simulink model "siso_4_channel_teleop_discrete_wave_forcePos_noise"  (R2021a)
settings: Solver=FixedStepAuto  StartTime=0.0  StopTime=30  FixedStep=Ts  RelTol=1e-3
values from neighbouring files (symbols this model uses):
  A_kalman = [1 Ts ; 0 1 ]    [assignment6.m]
  Amplitude = 1    [assignment6.m]
  b = 1    [assignment6.m]    (also in lessonParams.m)
  Be = 10    [assignment6.m]    (also in lessonParams.m)
  Bh = 1.5    [assignment6.m]    (also in lessonParams.m)
  Bs = 30    [assignment6.m]
  C_kalman = [1 0]    [assignment6.m]
  delay = 20    [assignment6.m]
  Dh = 2    [assignment6.m]    (also in lessonParams.m)
  Dm = 0    [assignment6.m]
  Ds = 0    [assignment6.m]
  Fc = 0.1    [assignment6.m]    (also in lessonParams.m = 1)
  Flp = 5    [assignment6.m]
  Ih = 0    [assignment6.m]
  Jh = 0    [assignment6.m]    (also in lessonParams.m = 0.05)
  k_h = 2    [assignment6.m]
  Ke = 200    [assignment6.m]    (also in lessonParams.m)
  Kh = 1    [assignment6.m]    (also in lessonParams.m = 0)
  Ks = 40    [assignment6.m]
  Mm = 0.5    [assignment6.m]
  Ms = 2    [assignment6.m]
  noiseVariance = 0.00001    (= 1e-05)    [assignment6.m]
  R = 1    [assignment6.m]
  Ts = 0.001    [assignment6.m]    (also in lessonParams.m)
  xe = 0.65    [assignment6.m]
undefined symbols (not defined in the file or in its folder): B, D, DiscIntNeverNeededParam, Discrete, Time
libraries: simulink x6, ctrlSharedLib x4
settings Model: Creator=fabio  LastModifiedBy=fabio

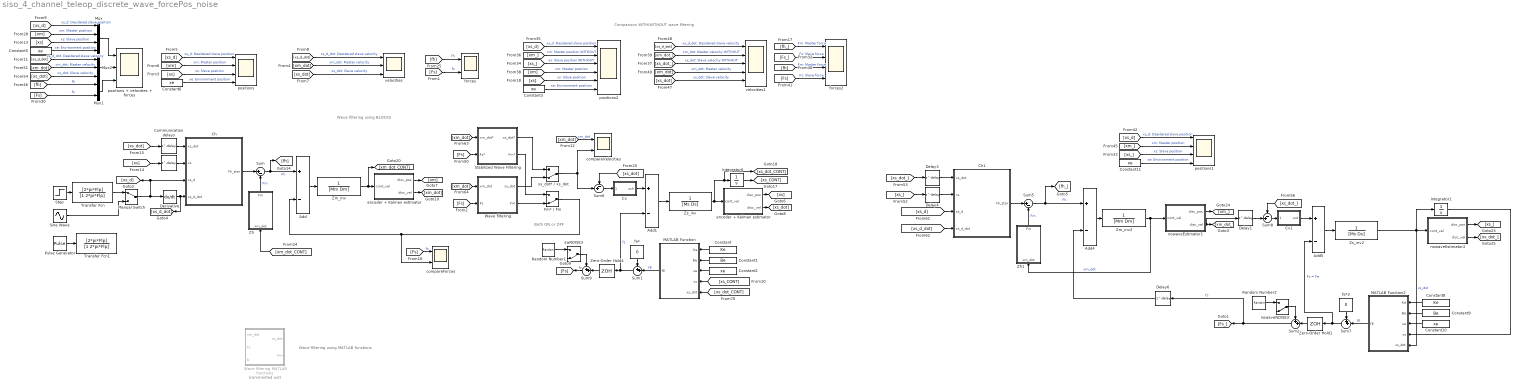
== system siso_4_channel_teleop_discrete_wave_forcePos_noise ==
  note: Both ON or OFF
  note: Wave filtering using BLOCKS
  note: Comparison WITH/WITHOUT wave filtering
  note: Wave filtering using MATLAB functions
  " " : Delay  DelayLength=delay  SampleTime=Ts
  Add{,1,4..5} (4 alike) : Sum  Inputs=+-
  Ch : Subsystem
  Ch1 : Subsystem
  Communication delays : Delay  DelayLength=delay  SampleTime=Ts
  Constant : Constant  Value=Ke
  Constant1 : Constant  Value=Be
  Constant{2..3,5..6,10..11} (6 alike) : Constant  Value=xe
  Constant8 : Constant  Value=Ke
  Constant9 : Constant  Value=Be
  Cv : Subsystem
  Cv1 : Subsystem
  Delay{1,3..4,6} (4 alike) : Delay  DelayLength=delay  SampleTime=Ts
  Derivative : Derivative
  Fm* / Fm : ManualSwitch  CurrentSetting=0
  Integrator1 : Integrator
  Integrator6 : Integrator
  MATLAB Function : MATLAB Function  TreatAsAtomicUnit=on
  MATLAB Function2 : MATLAB Function  TreatAsAtomicUnit=on
  Manual Switch : ManualSwitch
  Mux : Mux
  Mux1 : Mux  Inputs=2
  Mux2 : Mux  Inputs=3
  Pulse Generator : DiscretePulseGenerator  PulseType=Time based  Amplitude=Amplitude  PulseWidth=50  PhaseDelay=1
  Random Number1 : RandomNumber  Variance=noiseVariance  SampleTime=Ts
  Random Number2 : RandomNumber  Variance=noiseVariance  SampleTime=Ts
  Sine Wave : Sin  Amplitude=Amplitude  Frequency=Fc*2*pi  SampleTime=0
  Stabilized Wave Filtering : Subsystem
  Step : Step  After=Amplitude  SampleTime=0
  Sum : Sum  Inputs=|+-
  Sum{1..2,7,9} (4 alike) : Sum  Inputs=++|
  Sum5 : Sum  Inputs=|+-
  Sum6 : Sum  Inputs=-+|
  Sum8 : Sum  Inputs=-+|
  Transfer Fcn : TransferFcn  Numerator=[2*pi*Flp]  Denominator=[1 2*pi*Flp]
  Transfer Fcn1 : TransferFcn  Numerator=[2*pi*Flp]  Denominator=[1 2*pi*Flp]
  Wave filtering : Subsystem
  Wave filtering MATLAB functions : Subsystem  Commented=on
  Zero-Order Hold1 : ZeroOrderHold  SampleTime=Ts
  Zero-Order Hold4 : ZeroOrderHold  SampleTime=Ts
  Zh : Subsystem
  Zh1 : Subsystem
  Zm_inv : TransferFcn  Numerator=[0 1]  Denominator=[Mm Dm]
  Zm_inv2 : TransferFcn  Numerator=[0 1]  Denominator=[Mm Dm]
  Zs_inv : TransferFcn  Numerator=[0 1]  Denominator=[Ms Ds]
  Zs_inv2 : TransferFcn  Numerator=[0 1]  Denominator=[Ms Ds]
  compareForces : Scope  NumInputPorts=2
  compareVelocities : Scope  NumInputPorts=2
  encoder + Kalman estimator : Subsystem
  "encoder + Kalman estimator " : Subsystem
  fe* : Constant  Value=0
  fe*2 : Constant  Value=0
  forces : Scope  NumInputPorts=2
  forces2 : Scope  NumInputPorts=4
  nowaveEstimator1 : Subsystem
  nowaveEstimator2 : Subsystem
  nowaveNOISE3 : ManualSwitch  CurrentSetting=0
  positions : Scope  NumInputPorts=4
  positions + velocities + forces : Scope  NumInputPorts=3
  positions1 : Scope  NumInputPorts=4
  positions2 : Scope  NumInputPorts=6
  swNOISE3 : ManualSwitch  CurrentSetting=0
  velocities : Scope  NumInputPorts=3
  velocities1 : Scope  NumInputPorts=5
  xs_dot* / xs_dot : ManualSwitch  CurrentSetting=0
  wires:
  Zh/1(Fm) -> Sum/2  "Fm"
  Sum/1 -> Add/1, [fh]  "Fh"
  Constant/1 -> MATLAB Function/1(Ke)
  Constant1/1 -> MATLAB Function/2(Be)
  Constant2/1 -> MATLAB Function/3(xe)
  [xs_CONT] -> MATLAB Function/4(xs)
  [xs_dot_CONT] -> MATLAB Function/5(xs_dot)
  MATLAB Function/1(fE) -> Sum1/2  "fE"
  Cv/1(out) -> Add1/1
  Ch/1(Fh_star) -> Sum/1
  [xs_d] -> positions/1  "xs_d: Desidered slave position"
  [xm] -> positions/2  "xm: Master position"
  [xs] -> positions/3  "xs: Slave position"
  [xm_dot] -> velocities/2  "xm_dot: Master velocity"
  [xs_dot] -> velocities/3  "xs_dot: Slave velocity"
  [xs_d_dot] -> velocities/1  "xs_d_dot: Desidered slave velocity"
  Sine Wave/1 -> Manual Switch/2
  Derivative/1 -> [xs_d_dot], Ch/1(xs_d_dot)
  fe*/1 -> Sum1/1
  Step/1 -> Transfer Fcn/1
  Transfer Fcn/1 -> Manual Switch/1
  Manual Switch/1 -> Ch/2(xs_d), [xs_d], Derivative/1
  Constant6/1 -> positions/4  "xe: Environment position"
  [fh] -> forces/1  "fh"
  [Fs] -> forces/2  "fs"
  Pulse Generator/1 -> Transfer Fcn1/1
  [xs_dot] -> Communication delays/1
  Communication delays/1 -> Ch/4(xs_dot)
  " "/1 -> Ch/3(xs)
  [xs_dot] -> Sum6/1
  Sum6/1 -> Cv/1(velErr)
  Wave filtering/1(xs_dot) -> xs_dot* / xs_dot/2
  [Fs] -> Wave filtering/2(Fs)
  [xm_dot] -> compareVelocities/1  "xm_dot"
  [Fs] -> compareForces/1  "fs"
  [xs_d_dot] -> velocities1/1  "xs_d_dot: Desidered slave velocity"
  [xs_dot] -> velocities1/5  "xs_dot: Slave velocity"
  [fh_] -> forces2/1  "Fm: Master force"
  [xs_dot_] -> velocities1/3  "xs_dot: Slave velocity WITHOUT"
  [xm_dot_] -> velocities1/2  "xm_dot: Master velocity WITHOUT"
  [fh] -> forces2/3  "Fm: Master force"
  [xs] -> positions2/5  "xs: Slave position"
  [xs_d] -> positions2/1  "xs_d: Desidered slave position"
  [xm_dot] -> velocities1/4  "xm_dot: Master velocity"
  [Fs_] -> forces2/2  "Fs: Slave force"
  [xs_] -> positions2/3  "xs: Slave position WITHOUT"
  [xm] -> positions2/4  "xm: Master position"
  [xm_] -> positions2/2  "xm: Master position WITHOUT"
  Sum8/1 -> Cv1/1(velErr)
  [xs_dot_] -> Delay3/1
  fe*2/1 -> Sum7/1
  Delay3/1 -> Ch1/4(xs_dot)
  [xs_] -> Delay4/1
  [xs_dot_] -> Sum8/1
  Zh1/1(Fm) -> Sum5/2  "Fm"
  Zm_inv2/1 -> nowaveEstimator1/1(cont_vel), Zh1/1(xm_dot)  "xm_dot"
  Delay4/1 -> Ch1/3(xs)
  Constant9/1 -> MATLAB Function2/2(Be)
  Cv1/1(out) -> Add5/1
  Ch1/1(Fh_star) -> Sum5/1
  MATLAB Function2/1(fE) -> Sum7/2  "fE"
  Add5/1 -> Zs_inv2/1
  Constant10/1 -> MATLAB Function2/3(xe)
  Add4/1 -> Zm_inv2/1
  Constant8/1 -> MATLAB Function2/1(Ke)
  [xs_d] -> Ch1/2(xs_d)
  [xs_d_dot] -> Ch1/1(xs_d_dot)
  Sum5/1 -> [fh_], Add4/1  "Fh"
  [Fs] -> forces2/4  "Fs: Slave force"
  Constant11/1 -> positions1/4  "xe: Environment position"
  [xs_] -> positions1/3  "xs: Slave position"
  [xm_] -> positions1/2  "xm: Master position"
  [xs_d] -> positions1/1  "xs_d: Desidered slave position"
  Delay6/1 -> Add4/2
  nowaveEstimator1/2(disc_vel) -> Delay1/1, [xm_dot_]
  [Fs] -> Stabilized Wave Filtering/2(Fs*)
  xs_dot* / xs_dot/1 -> compareVelocities/2, Sum6/2
  Wave filtering/2(Fm) -> Fm* / Fm/2
  Sum1/1 -> Zero-Order Hold4/1, Add1/2  "fs"
  Zm_inv/1 -> [xm_dot_CONT], encoder + Kalman estimator/1(cont_vel)
  Integrator1/1 -> MATLAB Function2/4(xs)
  Fm* / Fm/1 -> compareForces/2, Add/2
  Zs_inv2/1 -> Integrator1/1, MATLAB Function2/5(xs_dot), nowaveEstimator2/1(cont_vel)  "xs_dot"
  [xm_dot] -> Stabilized Wave Filtering/1(xm_dot*)
  [xm_dot] -> Wave filtering/1(xm_dot)
  Add/1 -> Zm_inv/1
  encoder + Kalman estimator/2(disc_vel) -> [xm_dot]
  "encoder + Kalman estimator "/1(disc_pos) -> [xs]
  Zs_inv/1 -> "encoder + Kalman estimator "/1(cont_vel), [xs_dot_CONT], Integrator6/1
  Integrator6/1 -> [xs_CONT]
  Add1/1 -> Zs_inv/1
  encoder + Kalman estimator/1(disc_pos) -> [xm]
  [xm_dot_CONT] -> Zh/1(xm_dot)
  "encoder + Kalman estimator "/2(disc_vel) -> [xs_dot]
  Random Number1/1 -> swNOISE3/1
  swNOISE3/1 -> Sum9/1
  Sum9/1 -> [Fs]  "fs"
  Zero-Order Hold4/1 -> Sum9/2
  [xs] -> " "/1
  Stabilized Wave Filtering/1(xs_dot*) -> xs_dot* / xs_dot/1
  Stabilized Wave Filtering/2(Fm*) -> Fm* / Fm/1
  nowaveEstimator1/1(disc_pos) -> [xm_]
  nowaveEstimator2/2(disc_vel) -> [xs_dot_]
  nowaveEstimator2/1(disc_pos) -> [xs_]
  Zero-Order Hold1/1 -> Sum2/2
  nowaveNOISE3/1 -> Sum2/1
  Random Number2/1 -> nowaveNOISE3/1
  Sum7/1 -> Add5/2, Zero-Order Hold1/1  "Fs = Fe"
  Sum2/1 -> [Fs_], Delay6/1  "fs"
  Delay1/1 -> Sum8/2
  Constant3/1 -> positions2/6  "xe: Environment position"
  [Fs] -> Mux1/2  "fs"
  [xm] -> Mux/2  "xm: Master position"
  [xs_dot] -> Mux2/3  "xs_dot: Slave velocity"
  [xs] -> Mux/3  "xs: Slave position"
  [xm_dot] -> Mux2/2  "xm_dot: Master velocity"
  [fh] -> Mux1/1  "fh"
  [xs_d] -> Mux/1  "xs_d: Desidered slave position"
  Mux2/1 -> positions + velocities + forces/2
  Mux/1 -> positions + velocities + forces/1
  [xs_d_dot] -> Mux2/1  "xs_d_dot: Desidered slave velocity"
  Mux1/1 -> positions + velocities + forces/3
  Constant5/1 -> Mux/4  "xe: Environment position"

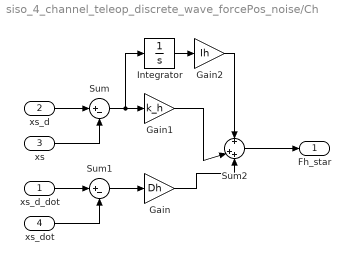
== system siso_4_channel_teleop_discrete_wave_forcePos_noise/Ch ==
  xs_d_dot : Inport
  xs_d : Inport  Port=2
  xs : Inport  Port=3
  xs_dot : Inport  Port=4
  Gain : Gain  Gain=Dh
  Gain1 : Gain  Gain=k_h
  Gain2 : Gain  Gain=Ih
  Integrator : Integrator
  Sum : Sum  Inputs=|+-
  Sum1 : Sum  Inputs=|+-
  Sum2 : Sum  Inputs=+|++
  Fh_star : Outport
  wires:
  Gain1/1 -> Sum2/2
  Sum2/1 -> Fh_star/1
  xs_d/1 -> Sum/1
  xs/1 -> Sum/2
  Sum/1 -> Integrator/1, Gain1/1
  xs_dot/1 -> Sum1/2
  Sum1/1 -> Gain/1
  Gain/1 -> Sum2/3
  xs_d_dot/1 -> Sum1/1
  Integrator/1 -> Gain2/1
  Gain2/1 -> Sum2/1

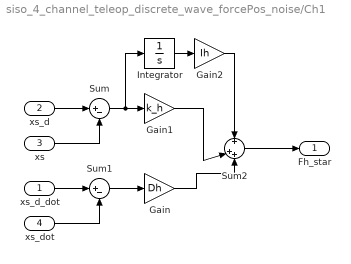
== system siso_4_channel_teleop_discrete_wave_forcePos_noise/Ch1 ==
  xs_d_dot : Inport
  xs_d : Inport  Port=2
  xs : Inport  Port=3
  xs_dot : Inport  Port=4
  Gain : Gain  Gain=Dh
  Gain1 : Gain  Gain=k_h
  Gain2 : Gain  Gain=Ih
  Integrator : Integrator
  Sum : Sum  Inputs=|+-
  Sum1 : Sum  Inputs=|+-
  Sum2 : Sum  Inputs=+|++
  Fh_star : Outport
  wires:
  Gain1/1 -> Sum2/2
  Sum2/1 -> Fh_star/1
  xs_d/1 -> Sum/1
  xs/1 -> Sum/2
  Sum/1 -> Integrator/1, Gain1/1
  xs_dot/1 -> Sum1/2
  Sum1/1 -> Gain/1
  Gain/1 -> Sum2/3
  xs_d_dot/1 -> Sum1/1
  Integrator/1 -> Gain2/1
  Gain2/1 -> Sum2/1

== system siso_4_channel_teleop_discrete_wave_forcePos_noise/Cv ==
  velErr : Inport
  Discrete-Time Integrator : DiscreteIntegrator  SampleTime=-1  ICPrevOutput=DiscIntNeverNeededParam  ICPrevScaledInput=DiscIntNeverNeededParam
  Gain : Gain  Gain=Bs
  Gain1 : Gain  Gain=Ks
  Manual Switch : ManualSwitch
  Sum : Sum  Inputs=|++
  out : Outport
  wires:
  velErr/1 -> Gain1/1, Manual Switch/1
  Gain1/1 -> Sum/1
  Sum/1 -> out/1
  Gain/1 -> Sum/2
  Manual Switch/1 -> Discrete-Time Integrator/1
  Discrete-Time Integrator/1 -> Gain/1

== system siso_4_channel_teleop_discrete_wave_forcePos_noise/Cv1 ==
  velErr : Inport
  Discrete-Time Integrator : DiscreteIntegrator  SampleTime=-1  ICPrevOutput=DiscIntNeverNeededParam  ICPrevScaledInput=DiscIntNeverNeededParam
  Gain : Gain  Gain=Bs
  Gain1 : Gain  Gain=Ks
  Manual Switch : ManualSwitch
  Sum : Sum  Inputs=|++
  out : Outport
  wires:
  velErr/1 -> Gain1/1, Manual Switch/1
  Gain1/1 -> Sum/1
  Sum/1 -> out/1
  Manual Switch/1 -> Gain/1
  Gain/1 -> Discrete-Time Integrator/1
  Discrete-Time Integrator/1 -> Sum/2

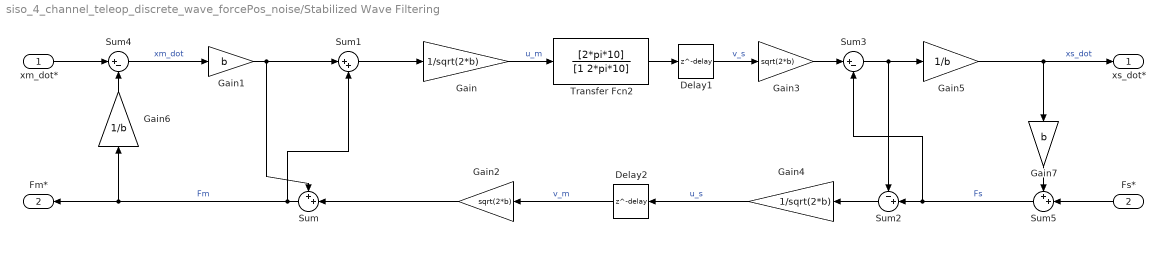
== system siso_4_channel_teleop_discrete_wave_forcePos_noise/Stabilized Wave Filtering ==
  xm_dot* : Inport
  Fs* : Inport  Port=2
  Delay1 : Delay  DelayLength=delay  SampleTime=Ts
  Delay2 : Delay  DelayLength=delay  SampleTime=Ts
  Gain : Gain  Gain=1/sqrt(2*b)
  Gain1 : Gain  Gain=b
  Gain2 : Gain  Gain=sqrt(2*b)
  Gain3 : Gain  Gain=sqrt(2*b)
  Gain4 : Gain  Gain=1/sqrt(2*b)
  Gain5 : Gain  Gain=1/b
  Gain6 : Gain  Gain=1/b
  Gain7 : Gain  Gain=b
  Sum : Sum  Inputs=++|
  Sum1 : Sum  Inputs=|++
  Sum2 : Sum  Inputs=-+|
  Sum3 : Sum  Inputs=|+-
  Sum4 : Sum  Inputs=|+-
  Sum5 : Sum  Inputs=++|
  Transfer Fcn2 : TransferFcn  Numerator=[2*pi*10]  Denominator=[1 2*pi*10]
  xs_dot* : Outport
  Fm* : Outport  Port=2
  wires:
  Delay1/1 -> Gain3/1  "v_s"
  Transfer Fcn2/1 -> Delay1/1
  Gain2/1 -> Sum/2
  Sum2/1 -> Gain4/1
  Gain/1 -> Transfer Fcn2/1  "u_m"
  Delay2/1 -> Gain2/1  "v_m"
  Gain3/1 -> Sum3/1
  Sum1/1 -> Gain/1
  Gain1/1 -> Sum/1, Sum1/1
  Sum3/1 -> Gain5/1, Sum2/1
  Gain4/1 -> Delay2/1  "u_s"
  Sum4/1 -> Gain1/1  "xm_dot"
  Gain6/1 -> Sum4/2
  xm_dot*/1 -> Sum4/1
  Sum/1 -> Sum1/2, Gain6/1, Fm*/1  "Fm"
  Gain7/1 -> Sum5/1
  Sum5/1 -> Sum3/2, Sum2/2  "Fs"
  Gain5/1 -> xs_dot*/1, Gain7/1  "xs_dot"
  Fs*/1 -> Sum5/2

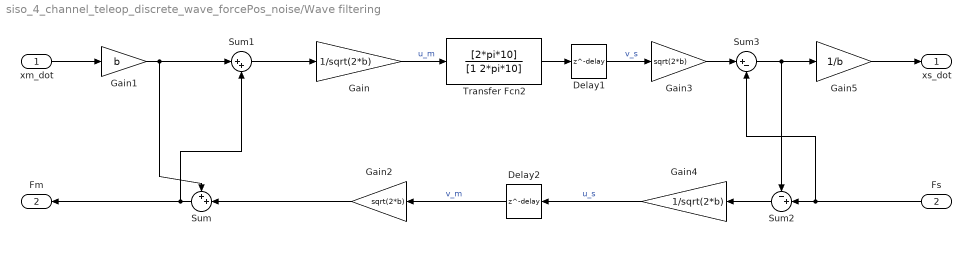
== system siso_4_channel_teleop_discrete_wave_forcePos_noise/Wave filtering ==
  xm_dot : Inport
  Fs : Inport  Port=2
  Delay1 : Delay  DelayLength=delay  SampleTime=Ts
  Delay2 : Delay  DelayLength=delay  SampleTime=Ts
  Gain : Gain  Gain=1/sqrt(2*b)
  Gain1 : Gain  Gain=b
  Gain2 : Gain  Gain=sqrt(2*b)
  Gain3 : Gain  Gain=sqrt(2*b)
  Gain4 : Gain  Gain=1/sqrt(2*b)
  Gain5 : Gain  Gain=1/b
  Sum : Sum  Inputs=++|
  Sum1 : Sum  Inputs=|++
  Sum2 : Sum  Inputs=-+|
  Sum3 : Sum  Inputs=|+-
  Transfer Fcn2 : TransferFcn  Numerator=[2*pi*10]  Denominator=[1 2*pi*10]
  xs_dot : Outport
  Fm : Outport  Port=2
  wires:
  Gain4/1 -> Delay2/1  "u_s"
  Sum3/1 -> Sum2/1, Gain5/1
  Gain1/1 -> Sum1/1, Sum/1
  Sum1/1 -> Gain/1
  Gain3/1 -> Sum3/1
  Delay2/1 -> Gain2/1  "v_m"
  Gain/1 -> Transfer Fcn2/1  "u_m"
  Sum2/1 -> Gain4/1
  Gain2/1 -> Sum/2
  xm_dot/1 -> Gain1/1
  Fs/1 -> Sum3/2, Sum2/2
  Sum/1 -> Fm/1, Sum1/2
  Gain5/1 -> xs_dot/1
  Transfer Fcn2/1 -> Delay1/1
  Delay1/1 -> Gain3/1  "v_s"

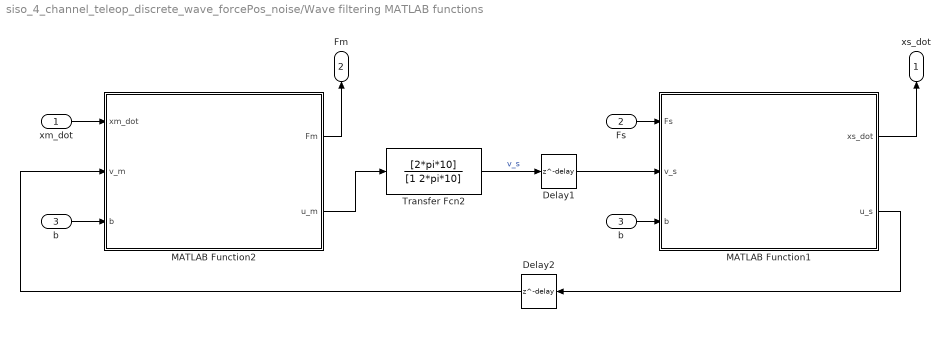
== system siso_4_channel_teleop_discrete_wave_forcePos_noise/Wave filtering MATLAB functions ==
  xm_dot : Inport
  Fs : Inport  Port=2
  b : Inport  Port=3
  Delay1 : Delay  DelayLength=delay  SampleTime=Ts
  Delay2 : Delay  DelayLength=delay  SampleTime=Ts
  MATLAB Function1 : MATLAB Function  TreatAsAtomicUnit=on
  MATLAB Function2 : MATLAB Function  TreatAsAtomicUnit=on
  Transfer Fcn2 : TransferFcn  Numerator=[2*pi*10]  Denominator=[1 2*pi*10]
  "b " : InportShadow  Port=3
  xs_dot : Outport
  Fm : Outport  Port=2
  wires:
  Transfer Fcn2/1 -> Delay1/1  "v_s"
  MATLAB Function1/2(u_s) -> Delay2/1
  Delay2/1 -> MATLAB Function2/2(v_m)
  b/1 -> MATLAB Function2/3(b)
  xm_dot/1 -> MATLAB Function2/1(xm_dot)
  "b "/1 -> MATLAB Function1/3(b)
  Delay1/1 -> MATLAB Function1/2(v_s)
  MATLAB Function1/1(xs_dot) -> xs_dot/1
  MATLAB Function2/1(Fm) -> Fm/1
  Fs/1 -> MATLAB Function1/1(Fs)
  MATLAB Function2/2(u_m) -> Transfer Fcn2/1

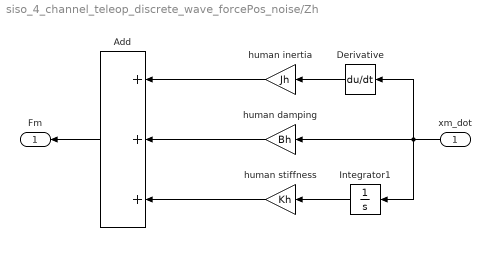
== system siso_4_channel_teleop_discrete_wave_forcePos_noise/Zh ==
  xm_dot : Inport
  Add : Sum  Inputs=+++
  Derivative : Derivative
  Integrator1 : Integrator
  human damping : Gain  Gain=Bh
  human inertia : Gain  Gain=Jh
  human stiffness : Gain  Gain=Kh
  Fm : Outport
  wires:
  Add/1 -> Fm/1
  human stiffness/1 -> Add/3
  human damping/1 -> Add/2
  Integrator1/1 -> human stiffness/1
  xm_dot/1 -> Derivative/1, Integrator1/1, human damping/1
  human inertia/1 -> Add/1
  Derivative/1 -> human inertia/1

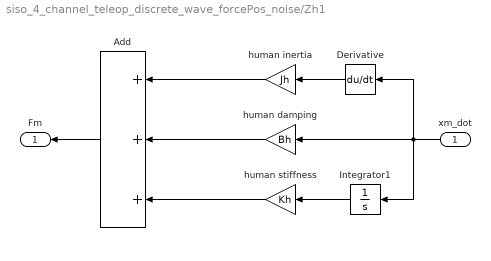
== system siso_4_channel_teleop_discrete_wave_forcePos_noise/Zh1 ==
  xm_dot : Inport
  Add : Sum  Inputs=+++
  Derivative : Derivative
  Integrator1 : Integrator
  human damping : Gain  Gain=Bh
  human inertia : Gain  Gain=Jh
  human stiffness : Gain  Gain=Kh
  Fm : Outport
  wires:
  Add/1 -> Fm/1
  human stiffness/1 -> Add/3
  human damping/1 -> Add/2
  Integrator1/1 -> human stiffness/1
  xm_dot/1 -> Derivative/1, Integrator1/1, human damping/1
  human inertia/1 -> Add/1
  Derivative/1 -> human inertia/1

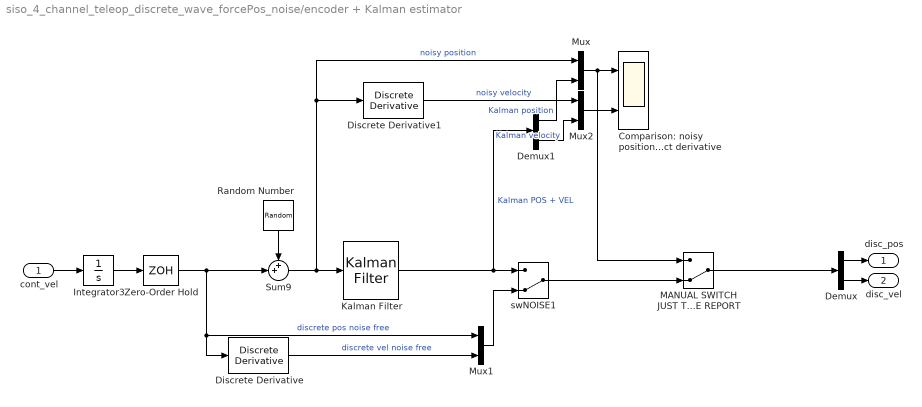
== system siso_4_channel_teleop_discrete_wave_forcePos_noise/encoder + Kalman estimator ==
  cont_vel : Inport
  Comparison: noisy position + Kalman/Direct derivative : Scope  NumInputPorts=2
  Demux : Demux  Outputs=2
  Demux1 : Demux  Outputs=2
  Discrete Derivative : simulink/Discrete/Discrete Derivative  gainval=1.0  ICPrevScaledInput=0.0  OutMin=[]  OutMax=[]  OutDataType=fixdt(1, 16)  OutScaling=2^-10  DoSatur=off
  Discrete Derivative1 : simulink/Discrete/Discrete Derivative  gainval=1.0  ICPrevScaledInput=0.0  OutMin=[]  OutMax=[]  OutDataType=fixdt(1, 16)  OutScaling=2^-10  DoSatur=off
  Integrator3 : Integrator
  Kalman Filter : ctrlSharedLib/Kalman Filter  TimeDomain=Discrete-Time  UseCurrentEstimator=on  ModelSource=Individual A, B, C, D matrices  ModelSourceVariable=sys  A=A_kalman  B=B  C=C_kalman  D=D  NumberOfStates=2  NumberOfInputs=2  NumberOfOutputs=2  InitialEstimateSource=Dialog  X0=0  P0=10  UseK=off  UseGH=off  NumberOfProcessNoiseInputs=2  G=1  TimeInvariantG=on  H=0  TimeInvariantH=on  Q=Q_master  TimeInvariantQ=on  R=R  TimeInvariantR=on  N=0  TimeInvariantN=on  AddInputPort=off  AddEnablePort=off  OutputEstimatedY=off  OutputP=off  Ts=Ts
  MANUAL SWITCH JUST TO PUT INSIDE REPORT : ManualSwitch  CurrentSetting=0
  Mux : Mux  Inputs=2
  Mux1 : Mux  Inputs=2
  Mux2 : Mux  Inputs=2
  Random Number : RandomNumber  Variance=noiseVariance  SampleTime=Ts
  Sum9 : Sum  Inputs=++|
  Zero-Order Hold : ZeroOrderHold  SampleTime=Ts
  swNOISE1 : ManualSwitch  CurrentSetting=0
  disc_pos : Outport
  disc_vel : Outport  Port=2
  wires:
  Integrator3/1 -> Zero-Order Hold/1
  cont_vel/1 -> Integrator3/1
  Random Number/1 -> Sum9/1
  Zero-Order Hold/1 -> Discrete Derivative/1, Mux1/1, Sum9/2  "discrete pos noise free"
  Demux/1 -> disc_pos/1
  Demux/2 -> disc_vel/1
  Discrete Derivative/1 -> Mux1/2  "discrete vel noise free"
  Mux1/1 -> swNOISE1/2
  Mux/1 -> MANUAL SWITCH JUST TO PUT INSIDE REPORT/1, Comparison: noisy position + Kalman/Direct derivative/1
  Demux1/2 -> Mux2/2  "Kalman velocity"
  Discrete Derivative1/1 -> Mux2/1  "noisy velocity"
  Kalman Filter/1 -> Demux1/1, swNOISE1/1  "Kalman POS + VEL"
  Sum9/1 -> Mux/1, Discrete Derivative1/1, Kalman Filter/1  "noisy position"
  Demux1/1 -> Mux/2  "Kalman position"
  Mux2/1 -> Comparison: noisy position + Kalman/Direct derivative/2
  MANUAL SWITCH JUST TO PUT INSIDE REPORT/1 -> Demux/1
  swNOISE1/1 -> MANUAL SWITCH JUST TO PUT INSIDE REPORT/2

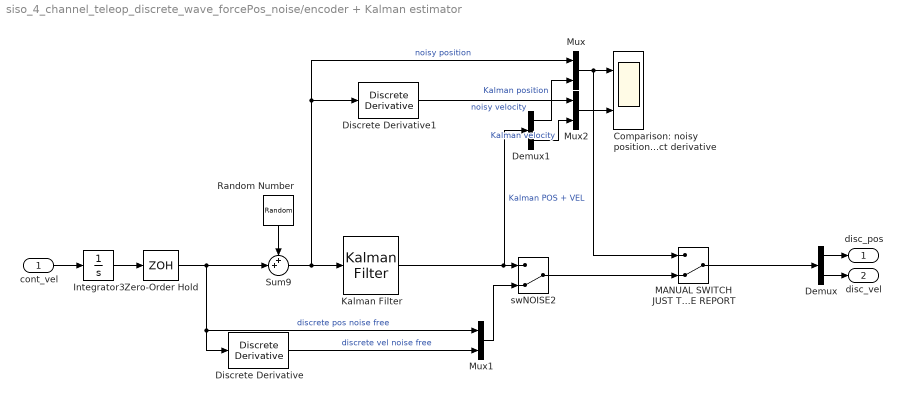
== system siso_4_channel_teleop_discrete_wave_forcePos_noise/encoder + Kalman estimator  ==
  cont_vel : Inport
  Comparison: noisy position + Kalman/Direct derivative : Scope  NumInputPorts=2
  Demux : Demux  Outputs=2
  Demux1 : Demux  Outputs=2
  Discrete Derivative : simulink/Discrete/Discrete Derivative  gainval=1.0  ICPrevScaledInput=0.0  OutMin=[]  OutMax=[]  OutDataType=fixdt(1, 16)  OutScaling=2^-10  DoSatur=off
  Discrete Derivative1 : simulink/Discrete/Discrete Derivative  gainval=1.0  ICPrevScaledInput=0.0  OutMin=[]  OutMax=[]  OutDataType=fixdt(1, 16)  OutScaling=2^-10  DoSatur=off
  Integrator3 : Integrator
  Kalman Filter : ctrlSharedLib/Kalman Filter  TimeDomain=Discrete-Time  UseCurrentEstimator=on  ModelSource=Individual A, B, C, D matrices  ModelSourceVariable=sys  A=A_kalman  B=B  C=C_kalman  D=D  NumberOfStates=2  NumberOfInputs=2  NumberOfOutputs=2  InitialEstimateSource=Dialog  X0=0  P0=10  UseK=off  UseGH=off  NumberOfProcessNoiseInputs=2  G=1  TimeInvariantG=on  H=0  TimeInvariantH=on  Q=Q_master  TimeInvariantQ=on  R=R  TimeInvariantR=on  N=0  TimeInvariantN=on  AddInputPort=off  AddEnablePort=off  OutputEstimatedY=off  OutputP=off  Ts=Ts
  MANUAL SWITCH JUST TO PUT INSIDE REPORT : ManualSwitch  CurrentSetting=0
  Mux : Mux  Inputs=2
  Mux1 : Mux  Inputs=2
  Mux2 : Mux  Inputs=2
  Random Number : RandomNumber  Variance=noiseVariance  SampleTime=Ts
  Sum9 : Sum  Inputs=++|
  Zero-Order Hold : ZeroOrderHold  SampleTime=Ts
  swNOISE2 : ManualSwitch  CurrentSetting=0
  disc_pos : Outport
  disc_vel : Outport  Port=2
  wires:
  Integrator3/1 -> Zero-Order Hold/1
  cont_vel/1 -> Integrator3/1
  Random Number/1 -> Sum9/1
  Zero-Order Hold/1 -> Discrete Derivative/1, Mux1/1, Sum9/2  "discrete pos noise free"
  Sum9/1 -> Mux/1, Discrete Derivative1/1, Kalman Filter/1  "noisy position"
  Kalman Filter/1 -> swNOISE2/1, Demux1/1  "Kalman POS + VEL"
  Demux/1 -> disc_pos/1
  Demux/2 -> disc_vel/1
  Discrete Derivative/1 -> Mux1/2  "discrete vel noise free"
  Mux1/1 -> swNOISE2/2
  Mux/1 -> MANUAL SWITCH JUST TO PUT INSIDE REPORT/1, Comparison: noisy position + Kalman/Direct derivative/1
  Demux1/1 -> Mux/2  "Kalman position"
  Mux2/1 -> Comparison: noisy position + Kalman/Direct derivative/2
  Discrete Derivative1/1 -> Mux2/1  "noisy velocity"
  Demux1/2 -> Mux2/2  "Kalman velocity"
  MANUAL SWITCH JUST TO PUT INSIDE REPORT/1 -> Demux/1
  swNOISE2/1 -> MANUAL SWITCH JUST TO PUT INSIDE REPORT/2

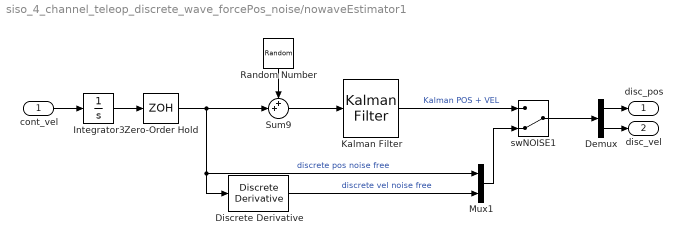
== system siso_4_channel_teleop_discrete_wave_forcePos_noise/nowaveEstimator1 ==
  cont_vel : Inport
  Demux : Demux  Outputs=2
  Discrete Derivative : simulink/Discrete/Discrete Derivative  gainval=1.0  ICPrevScaledInput=0.0  OutMin=[]  OutMax=[]  OutDataType=fixdt(1, 16)  OutScaling=2^-10  DoSatur=off
  Integrator3 : Integrator
  Kalman Filter : ctrlSharedLib/Kalman Filter  TimeDomain=Discrete-Time  UseCurrentEstimator=on  ModelSource=Individual A, B, C, D matrices  ModelSourceVariable=sys  A=A_kalman  B=B  C=C_kalman  D=D  NumberOfStates=2  NumberOfInputs=2  NumberOfOutputs=2  InitialEstimateSource=Dialog  X0=0  P0=10  UseK=off  UseGH=off  NumberOfProcessNoiseInputs=2  G=1  TimeInvariantG=on  H=0  TimeInvariantH=on  Q=Q_master  TimeInvariantQ=on  R=R  TimeInvariantR=on  N=0  TimeInvariantN=on  AddInputPort=off  AddEnablePort=off  OutputEstimatedY=off  OutputP=off  Ts=Ts
  Mux1 : Mux  Inputs=2
  Random Number : RandomNumber  Variance=noiseVariance  SampleTime=Ts
  Sum9 : Sum  Inputs=++|
  Zero-Order Hold : ZeroOrderHold  SampleTime=Ts
  swNOISE1 : ManualSwitch  CurrentSetting=0
  disc_pos : Outport
  disc_vel : Outport  Port=2
  wires:
  Integrator3/1 -> Zero-Order Hold/1
  cont_vel/1 -> Integrator3/1
  Random Number/1 -> Sum9/1
  Zero-Order Hold/1 -> Discrete Derivative/1, Mux1/1, Sum9/2  "discrete pos noise free"
  Sum9/1 -> Kalman Filter/1
  Kalman Filter/1 -> swNOISE1/1  "Kalman POS + VEL"
  swNOISE1/1 -> Demux/1
  Demux/1 -> disc_pos/1
  Demux/2 -> disc_vel/1
  Discrete Derivative/1 -> Mux1/2  "discrete vel noise free"
  Mux1/1 -> swNOISE1/2

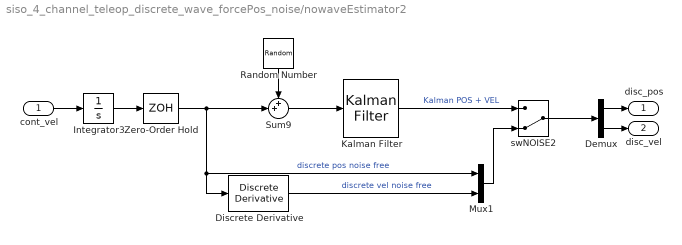
== system siso_4_channel_teleop_discrete_wave_forcePos_noise/nowaveEstimator2 ==
  cont_vel : Inport
  Demux : Demux  Outputs=2
  Discrete Derivative : simulink/Discrete/Discrete Derivative  gainval=1.0  ICPrevScaledInput=0.0  OutMin=[]  OutMax=[]  OutDataType=fixdt(1, 16)  OutScaling=2^-10  DoSatur=off
  Integrator3 : Integrator
  Kalman Filter : ctrlSharedLib/Kalman Filter  TimeDomain=Discrete-Time  UseCurrentEstimator=on  ModelSource=Individual A, B, C, D matrices  ModelSourceVariable=sys  A=A_kalman  B=B  C=C_kalman  D=D  NumberOfStates=2  NumberOfInputs=2  NumberOfOutputs=2  InitialEstimateSource=Dialog  X0=0  P0=10  UseK=off  UseGH=off  NumberOfProcessNoiseInputs=2  G=1  TimeInvariantG=on  H=0  TimeInvariantH=on  Q=Q_master  TimeInvariantQ=on  R=R  TimeInvariantR=on  N=0  TimeInvariantN=on  AddInputPort=off  AddEnablePort=off  OutputEstimatedY=off  OutputP=off  Ts=Ts
  Mux1 : Mux  Inputs=2
  Random Number : RandomNumber  Variance=noiseVariance  SampleTime=Ts
  Sum9 : Sum  Inputs=++|
  Zero-Order Hold : ZeroOrderHold  SampleTime=Ts
  swNOISE2 : ManualSwitch  CurrentSetting=0
  disc_pos : Outport
  disc_vel : Outport  Port=2
  wires:
  Integrator3/1 -> Zero-Order Hold/1
  cont_vel/1 -> Integrator3/1
  Random Number/1 -> Sum9/1
  Zero-Order Hold/1 -> Discrete Derivative/1, Mux1/1, Sum9/2  "discrete pos noise free"
  Sum9/1 -> Kalman Filter/1
  Kalman Filter/1 -> swNOISE2/1  "Kalman POS + VEL"
  swNOISE2/1 -> Demux/1
  Demux/1 -> disc_pos/1
  Demux/2 -> disc_vel/1
  Discrete Derivative/1 -> Mux1/2  "discrete vel noise free"
  Mux1/1 -> swNOISE2/2

== matlab function siso_4_channel_teleop_discrete_wave_forcePos_noise/MATLAB Function ==
  data: Ke input; fE output; Be input; xe input; xs input; xs_dot input
function fE = environment(Ke, Be, xe, xs, xs_dot)
    if xs > xe
        fE = Ke*(xs - xe) + Be*xs_dot;
    else
        fE = 0;
    end
end

== matlab function siso_4_channel_teleop_discrete_wave_forcePos_noise/MATLAB Function2 ==
  data: Ke input; fE output; Be input; xe input; xs input; xs_dot input
function fE = environment(Ke, Be, xe, xs, xs_dot)
    if xs > xe
        fE = Ke*(xs - xe) + Be*xs_dot;
    else
        fE = 0;
    end
end

== matlab function siso_4_channel_teleop_discrete_wave_forcePos_noise/Wave filtering MATLAB functions/MATLAB Function1 ==
  data: Fs input; xs_dot output; v_s input; u_s output; b input
function [xs_dot, u_s] = wave_fromTo_power_R(Fs, v_s, b)

    xs_dot = 1/b*( -Fs + sqrt(2*b)*v_s );
%     u_s  = 1/sqrt(2*b)*( -b*xs_dot + Fs ); %the same
    u_s  = 1/sqrt(2*b)*( Fs - (v_s*sqrt(2*b)-Fs) );

end

== matlab function siso_4_channel_teleop_discrete_wave_forcePos_noise/Wave filtering MATLAB functions/MATLAB Function2 ==
  data: xm_dot input; Fm output; v_m input; u_m output; b input
function [Fm, u_m] = wave_fromTo_power_L(xm_dot, v_m, b)
    
    Fm = b*xm_dot + sqrt(2*b)*v_m;
    u_m  = 1/sqrt(2*b) * (b*xm_dot + Fm);
    
end
